simulink model "s433a"  (Simulink 5.1)
settings: Solver=ode45  StartTime=0.0  StopTime=100.0  RelTol=1e-3
settings Model: LastModifiedBy=user_father  BooleanDataType=on  ProdHWDeviceType=Microprocessor

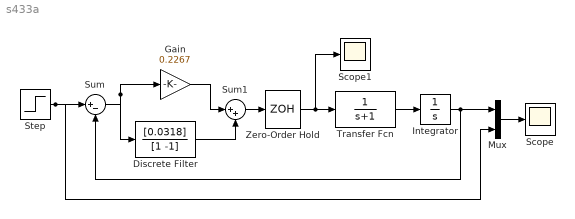
== system s433a ==
  Discrete Filter : DiscreteFilter  Numerator=[0.0318]  Denominator=[1 -1]
  Gain : Gain  Gain=0.2267  SaturateOnIntegerOverflow=on
  Integrator : Integrator
  Mux : Mux  Inputs=2
  Scope : Scope
  Scope1 : Scope
  Step : Step  Time=0  SampleTime=0
  Sum : Sum  Inputs=|+-  SaturateOnIntegerOverflow=on
  Sum1 : Sum  Inputs=|++  SaturateOnIntegerOverflow=on
  Transfer Fcn : TransferFcn  Denominator=[1 1]
  Zero-Order Hold : ZeroOrderHold
  wires:
  Transfer Fcn/1 -> Integrator/1
  Zero-Order Hold/1 -> Scope1/1, Transfer Fcn/1
  Step/1 -> Sum/1, Mux/2
  Sum/1 -> Gain/1, Discrete Filter/1
  Sum1/1 -> Zero-Order Hold/1
  Discrete Filter/1 -> Sum1/2
  Gain/1 -> Sum1/1
  Mux/1 -> Scope/1
  Integrator/1 -> Mux/1, Sum/2
